simulink model "Diag_Etat_Test_Roomba2"  (R2015b)
settings: Solver=VariableStepAuto  StartTime=0.0  StopTime=inf  FixedStep=1  RelTol=1e-3
InitFcn:
  | iRobotControl_switchyard('setup_localPCclock');iRobotControl_switchyard('setup_StarGazer_landmark_offset_table')
undefined symbols (not defined in the file or in its folder): iRobotControl_switchyard
libraries: realtime_pacer_lib x1
CloseFcn:
  | iRobotControl_switchyard close_iRobotControl
settings Model: Creator=sksu  LastModifiedBy=Sebastien
settings DataIOCC: SaveFormat=Array  SignalLoggingSaveFormat=ModelDataLogs
settings OptimizationCC: ExpressionDepthLimit=2147483647
settings DebuggingCC: UnderspecifiedInitializationDetection=Classic  MergeDetectMultiDrivingBlocksExec=none  SolverPrmCheckMsg=warning  FcnCallInpInsideContextMsg=EnableAllAsWarning  StateNameClashWarn=warning
settings HardwareCC: ProdBitPerPointer=32  ProdLargestAtomicFloat=None  ProdIntDivRoundTo=Undefined  ProdEndianess=Unspecified  ProdWordSize=32  ProdHWDeviceType=32-bit Generic
settings GRTTargetCC: GeneratePreprocessorConditionals=Disable all
settings ConfigComp: CovModelRefEnable=Off

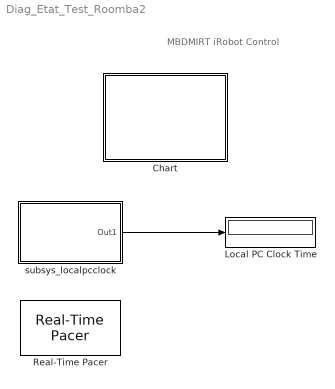
== system Diag_Etat_Test_Roomba2 ==
  note: MBDMIRT iRobot Control
  Chart : Stateflow chart  TreatAsAtomicUnit=on
  Local PC Clock Time : Display
  Real-Time Pacer : realtime_pacer_lib/Real-Time Pacer  simTimePerRealTime=1000
  subsys_localpcclock : Subsystem
      mask Display: fprintf('Elapsed Local PC\nClock')
  wires:
  subsys_localpcclock/1(Out1) -> Local PC Clock Time/1

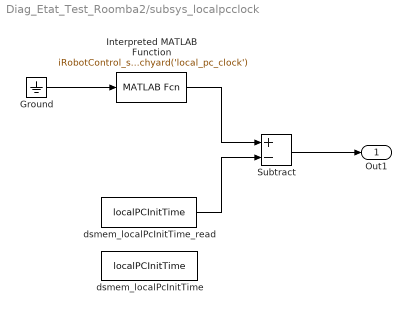
== system Diag_Etat_Test_Roomba2/subsys_localpcclock ==
  Ground : Ground
  Interpreted MATLAB Function : MATLABFcn  MATLABFcn=iRobotControl_switchyard('local_pc_clock')  OutputSignalType=real
  Subtract : Sum  Inputs=+-
  dsmem_localPcInitTime : DataStoreMemory  DataStoreName=localPCInitTime  WriteAfterWriteMsg=warning  WriteAfterReadMsg=warning  InitialValue=1543052.182  OutDataTypeStr=double
  dsmem_localPcInitTime_read : DataStoreRead  DataStoreName=localPCInitTime  SampleTime=1
  Out1 : Outport
  wires:
  Ground/1 -> Interpreted MATLAB Function/1
  Interpreted MATLAB Function/1 -> Subtract/1
  dsmem_localPcInitTime_read/1 -> Subtract/2
  Subtract/1 -> Out1/1

== stateflow chart Diag_Etat_Test_Roomba2/Chart ==
  settings: updateMethod=DISCRETE  sampleTime=1
  state AngleR = AngleSensorRoomba(serObjNum) [function]
    (default) -> (junction 640) : { AngleR = ml('AngleSensorRoomba(iRobot_%d)', serObjNum); }
  state clk = LocalPCClock [function]
    (default) -> (junction 1924) : {clk = ml.iRobotControl_switchyard('local_pc_clock');}
  state state = CliffRightSensorRoomba(serObjNum) [function]
    (default) -> (junction 756) : { state = ml('CliffRightSensorRoomba(iRobot_%d)', serObjNum); }
  state [Charge, Capacity, Percent] = BatteryChargeReaderRoomba(serObjNum) [function]
    (default) -> (junction 665) : {
        | /* Reset container for battery status */
        | ml('iRobot_%d_BattCharSensor(1:3)=0;', serObjNum);
        |
        | /* Read battery status */
        | ml('[iRobot_%d_BattCharSensor(1), iRobot_%d_BattCharSensor(2), iRobot_%d_BattCharSensor(3)]=BatteryChargeReaderRoomba(iRobot_%d);',...
        |       serObjNum, serObjNum, serObjNum, serObjNum);
        |
        |
        | BattCharSensor=ml('iRobot_%d_BattCharSensor', serObjNum);
        |
        | Charge=BattCharSensor[0];
        | Capacity=BattCharSensor[1];
        | Percent=BattCharSensor[2];
        | }
  state strg = CliffRightSignalStrengthRoomba(serObjNum) [function]
    (default) -> (junction 761) : { strg = ml('CliffRightSignalStrengthRoomba(iRobot_%d)', serObjNum); }
  state BeepRoomba(serObjNum) [function]
    (default) -> (junction 686) : { ml('BeepRoomba(iRobot_%d)', serObjNum); }
  state iRobot_Test
    state INIT
      en: irobotID=1;
      serObjNum=RoombaInit(irobotID);
    state DEPLACEMENT
      du:
      [Dock, Clean] = ButtonsSensorRoomba(serObjNum);
      state Fwd_Bwd
        state moveFwd_After5sec
          en: SetLCDRoomba(serObjNum, 97,98,99,0);
          SetFwdVelAngVelCreate(serObjNum, 0.05, 0);
          SetLEDsRoomba(serObjNum, 1, 0, 100);
          SetBrushRoomba(serObjNum, 1);
          seenClk=LocalPCClock();
          du:
          currClk=LocalPCClock();
        state moveBwd_After5sec
          en:  SetLCDRoomba(serObjNum, 0,97,98,99);
          SetFwdVelAngVelCreate(serObjNum, -0.05, 0);
          SetLEDsRoomba(serObjNum, 1, 100, 100);
          SetBrushRoomba(serObjNum, 9);
          seenClk=LocalPCClock();
          du:
          currClk=LocalPCClock();
        (default) -> moveFwd_After5sec
        moveFwd_After5sec -> moveBwd_After5sec : [currClk-seenClk>=5]
        moveBwd_After5sec -> moveFwd_After5sec : [currClk-seenClk>=5]
      state STOP
        en: SetFwdVelAngVelCreate(serObjNum, 0, 0);
        SetLEDsRoomba(serObjNum, 0, 10, 100);
        SetBrushRoomba(serObjNum, 0);
      Fwd_Bwd -> STOP : [Dock]
      STOP -> Fwd_Bwd : [Clean]
      (default) -> STOP
    INIT -> DEPLACEMENT
    (default) -> INIT
  state [BumpRight, BumpLeft, WheDropRight, WheDropLeft, ... [function]
    WheDropCaster, BumpFront] = BumpsWheelDropsSensorsRoomba(serObjNum)
    (default) -> (junction 455) : {
        | /* Reset container for bump and wheel sensors */
        | ml('iRobot_%d_BmpWhlSensor(1:6)=0;', serObjNum);
        |
        | /* Read bump and wheel sensors */
        | ml('[iRobot_%d_BmpWhlSensor(1), iRobot_%d_BmpWhlSensor(2), iRobot_%d_BmpWhlSensor(3), iRobot_%d_BmpWhlSensor(4), iRobot_%d_BmpWhlSensor(5), iRobot_%d_BmpWhlSensor(6)]=BumpsWheelDropsSensorsRoomba(iRobot_%d);',...
        |       serObjNum, serObjNum, serObjNum, serObjNum, serObjNum, serObjNum, serObjNum);
        |
        |
        | BmpWhlSensor = ml('iRobot_%d_BmpWhlSensor', serObjNum);
        |
        | BumpRight=BmpWhlSensor[0];
        | BumpLeft=BmpWhlSensor[1];
        | WheDropRight=BmpWhlSensor[2];
        | WheDropLeft=BmpWhlSensor[3];
        | WheDropCaster=BmpWhlSensor[4];
        | BumpFront=BmpWhlSensor[5];
        | }
  state Current = CurrentTesterRoomba(serObjNum) [function]
    (default) -> (junction 766) : { Current = ml('CurrentTesterRoomba(iRobot_%d)', serObjNum); }
  state [ButtonAdv, ButtonPlay] = ButtonsSensorRoomba(serObjNum) [function]
    (default) -> (junction 694) : {
        | /* Reset container for buttons seonsor */
        | ml('iRobot_%d_ButtSensor(1:2)=0;', serObjNum);
        |
        | /* Read battery status */
        | ml('[iRobot_%d_ButtSensor(1), iRobot_%d_ButtSensor(2)]=ButtonsSensorRoomba(iRobot_%d);',...
        |       serObjNum, serObjNum, serObjNum);
        |
        |
        | ButtSensor=ml('iRobot_%d_ButtSensor', serObjNum);
        |
        | ButtonAdv=ButtSensor[0];
        | ButtonPlay=ButtSensor[1];
        | }
  state Distance = DistanceSensorRoomba(serObjNum) [function]
    (default) -> (junction 801) : { Distance = ml('DistanceSensorRoomba(iRobot_%d)', serObjNum); }
  state state = CliffFrontLeftSensorRoomba(serObjNum) [function]
    (default) -> (junction 718) : { state = ml('CliffFrontLeftSensorRoomba(iRobot_%d)', serObjNum); }
  state serObjNum = RoombaInit(irobotID) [function]
    (default) -> (junction 574) : /* Check if expected variable exists*/
        | { flag_exist=ml('exist(''iRobot_%d'',''var'')', irobotID); }
    (junction 574) -> (junction 575) [order 1] : [ flag_exist==true ]
    (junction 575) -> (junction 580) : /* Check if the expected variable is a serial object */
        | { flag_serport=ml('isa(iRobot_%d, ''serial'')', irobotID); }
    (junction 574) -> (junction 578) [order 2]
    (junction 580) -> (junction 576) [order 1] : [ flag_serport==true ]
    (junction 580) -> (junction 577) [order 2]
    (junction 576) -> (junction 581) : { serObjNum=irobotID; }
    (junction 577) -> (junction 578)
    (junction 578) -> (junction 2272) : { ml.error('iRobot_%d is not initialized.', irobotID); }
  state strg = CliffFrontLeftSignalStrengthRoomba(serObjNum) [function]
    (default) -> (junction 729) : { strg = ml('CliffFrontLeftSignalStrengthRoomba(iRobot_%d)', serObjNum); }
  state SetDriveWheelsCreate(serObjNum, rightWheelVel, leftWheelVel) [function]
    (default) -> (junction 809) : { ml('SetDriveWheelsCreate(iRobot_%d, %f, %f)', serObjNum, rightWheelVel, leftWheelVel); }
  state state = CliffFrontRightSensorRoomba(serObjNum) [function]
    (default) -> (junction 736) : { state = ml('CliffFrontRightSensorRoomba(iRobot_%d)', serObjNum); }
  state SetFwdVelAngVelCreate(serObjNum, FwdVel, AngVel) [function]
    (default) -> (junction 65) : { ml('SetFwdVelAngVelCreate(iRobot_%d, %f, %f)', serObjNum, FwdVel, AngVel); }
  state SetBrushRoomba(serObjNum, Brushes) [function]
    (default) -> (junction 3475) : { ml('SetBrushRoomba(iRobot_%d, %f)', serObjNum, Brushes); }
  state SetFwdVelRadiusRoomba(serObjNum, FwdVel, Radius) [function]
    (default) -> (junction 816) : { ml('SetFwdVelRadiusRoomba(iRobot_%d, %f, %f)', serObjNum, FwdVel, Radius); }
  state strg = CliffFrontRightSignalStrengthRoomba(serObjNum) [function]
    (default) -> (junction 741) : { strg = ml('CliffFrontRightSignalStrengthRoomba(iRobot_%d)', serObjNum); }
  state SetLCDRoomba(serObjNum, D3,D2,D1,D0) [function]
    (default) -> (junction 3466) : { ml('SetLCDRoomba(iRobot_%d, %f, %f, %f, %f)', serObjNum, D3, D2, D1, D0); }
  state state = CliffLeftSensorRoomba(serObjNum) [function]
    (default) -> (junction 746) : { state = ml('CliffLeftSensorRoomba(iRobot_%d)', serObjNum); }
  state SetLEDsRoomba(serObjNum, LED,Color, Intensity) [function]
    (default) -> (junction 823) : { ml('SetLEDsRoomba(iRobot_%d, %f, %f, %f)', serObjNum, LED, Color, Intensity); }
  state strg = CliffLeftSignalStrengthRoomba(serObjNum) [function]
    (default) -> (junction 751) : { strg = ml('CliffLeftSignalStrengthRoomba(iRobot_%d)', serObjNum); }
  state travelDist(serObjNum, speed, distance) [function]
    (default) -> (junction 294) : { ml('travelDist(iRobot_%d, %f, %f)', serObjNum, speed, distance); }
  state turnAngle(serObjNum, speed, angle) [function]
    (default) -> (junction 335) : { ml('turnAngle(iRobot_%d, %f, %f)', serObjNum, speed, angle); }
  (default) -> iRobot_Test
  data: serObjNum function_input int16; AngleR function_output double; clk function_output double; serObjNum function_input int16; state function_output double; Charge function_output double; Capacity function_output double; Percent function_output double; serObjNum function_input int16; BattCharSensor temporary double size=1,3; serObjNum function_input int16; strg function_output double; serObjNum function_input int16; serObjNum local double; bR local double; bL local double; wR local double; wL local double; wCst local double; bF local double; ang_turned local double; irobotID local double; pi parameter double; currClk local double; seenClk local double; BumpRight function_output double; BumpLeft function_output double; WheDropRight function_output double; WheDropLeft function_output double; WheDropCaster function_output double; serObjNum function_input int16; BumpFront function_output double; BmpWhlSensor temporary double size=1,6; serObjNum function_input int16; Current function_output double; ButtonAdv function_output double; ButtonPlay function_output double; serObjNum function_input int16; ButtSensor temporary double size=1,2; Distance function_output double; serObjNum function_input int16; serObjNum function_input int16; state function_output double; irobotID function_input int16; serObjNum function_output int16; flag_serport temporary boolean; flag_exist temporary boolean; serObjNum function_input int16; strg function_output double; serObjNum function_input int16; rightWheelVel function_input double; leftWheelVel function_input double; serObjNum function_input int16; state function_output double; serObjNum function_input int16; FwdVel function_input double; AngVel function_input double; serObjNum function_input int16; Brushes function_input double; serObjNum function_input int16; FwdVel function_input double; Radius function_input double; serObjNum function_input int16; strg function_output double; serObjNum function_input int16; D3 function_input double; D2 function_input double; D1 function_input double; D0 function_input double; serObjNum function_input int16; state function_output double; serObjNum function_input int16; LED function_input double; Color function_input double; Intensity function_input double; serObjNum function_input int16; strg function_output double; serObjNum function_input int16; speed function_input double; distance function_input double; serObjNum function_input int16; speed function_input double; angle function_input double; cf_FL local double; cf_FR local double; fwdVel local double; irobotID local double; radi_L local double; radi_S local double; serObjNum local double; BumpLeft local double; BumpRight local double; WheDropCaster local double; WheDropLeft local double; WheDropRight local double; BumpFront local double; Dock local double; Clean local double
  events: ButtonClean local FUNCTION_CALL_EVENT; ButtonDock local FUNCTION_CALL_EVENT
